simulink model "Pend"  (Simulink 7.4)
settings: Solver=ode45  StartTime=0.0  StopTime=10.0  RelTol=1e-3
libraries: mblibv1 x10
settings Model: Creator=marsryu  LastModifiedBy=marsryu
settings SimMechanicsCC: VisOnUpdateDiagram=on  VisDuringSimulation=on

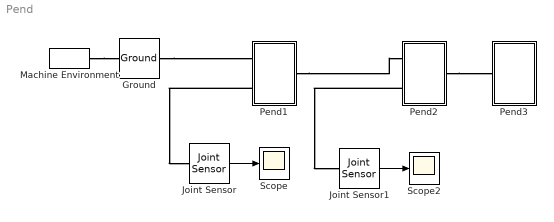
== system Pend ==
  Ground : mblibv1/Bodies/Ground  DialogController=MECH.DynMechDlgSource  SystemSampleTime=-1  UpdateFromCAD=off  LeftPortType=env  RightPortType=workingframe  PhysicalDomain=Mechanical  DialogClass=GroundBlock  CoordPosition=[0 0 0]  CoordPositionUnits=m  StateVectorMgrId=-1  MachineId=[0 0]  ShowEnvPort=on
  Joint Sensor : mblibv1/Sensors &  Actuators/Joint Sensor  DialogController=MECH.DynMechDlgSource  SystemSampleTime=-1  UpdateFromCAD=off  PhysicalDomain=Mechanical  PortType=blob  Muxed=off  Pose=off  Angle=on  AngleUnits=deg  ArcVelocity=off  ArcVelocityUnits=deg/s  ArcAcceleration=off  ArcAccelerationUnits=deg/s^2  CoordPosition=on  CoordPositionUnits=m  Velocity=off  VelocityUnits=m/s  Acceleration=off  AccelerationUnits=m/s^2  Quaternion=on  QuaternionDT=off  QuaternionDDT=off  QuaternionUnits=off  OutputVector=[1]  ActiveIO=on  Width=1  DialogClass=MechanicalSensorBlock  Primitive=R1  Force=off  ForceUnits=N  Torque=off  TorqueUnits=N*m  ReferenceFrame=Absolute (World)  ReactionSensedSide=Base  ReactionReferenceFrame=Absolute (World)  ReactionForce=off  ReactionForceUnits=N  ReactionMoment=off  ReactionMomentUnits=N*m
  Joint Sensor1 : mblibv1/Sensors &  Actuators/Joint Sensor  DialogController=MECH.DynMechDlgSource  SystemSampleTime=-1  UpdateFromCAD=off  PhysicalDomain=Mechanical  PortType=blob  Muxed=on  Pose=off  Angle=on  AngleUnits=deg  ArcVelocity=off  ArcVelocityUnits=deg/s  ArcAcceleration=off  ArcAccelerationUnits=deg/s^2  CoordPosition=on  CoordPositionUnits=m  Velocity=off  VelocityUnits=m/s  Acceleration=off  AccelerationUnits=m/s^2  Quaternion=on  QuaternionDT=off  QuaternionDDT=off  QuaternionUnits=off  OutputVector=[1]  ActiveIO=on  Width=1  DialogClass=MechanicalSensorBlock  Primitive=R1  Force=off  ForceUnits=N  Torque=off  TorqueUnits=N*m  ReferenceFrame=Absolute (World)  ReactionSensedSide=Base  ReactionReferenceFrame=Absolute (World)  ReactionForce=off  ReactionForceUnits=N  ReactionMoment=off  ReactionMomentUnits=N*m
  Machine Environment : mblibv1/Bodies/Machine Environment  DialogController=MECH.DialogSource  SystemSampleTime=-1  PortType=env  PhysicalDomain=Mechanical  DialogTemplateClass=MECH.MachineEnvironment  SyncWhenCopied=off  Gravity=[0 -9.81 0]  GravityUnits=m/s^2  GravityAsSignal=off  Dimensionality=Auto-detect  AnalysisType=Forward dynamics  LinearAssemblyTolerance=1e-3  LinearAssemblyToleranceUnits=m  AngularAssemblyTolerance=1e-3  AngularAssemblyToleranceUnits=rad  ConstraintSolverType=Stabilizing  ConstraintRelTolerance=1e-4  ConstraintAbsTolerance=1e-4  UseRobustSingularityHandling=off  RedundancyAnalysisToleranceType=Automatically select tolerance  RedundancyAnalysisTolerance=1e-14  StatePerturbationType=Fixed  PerturbationSize=1e-5  VisualizeMachine=on  BodyVisualizationType=Use model default body geometries  BodyColorSelMode=Use model default  DefaultBodyColor=[1 0 0]
  Pend1 : Subsystem
  Pend2 : Subsystem
  Pend3 : Subsystem
  Scope : Scope
  Scope2 : Scope
      settings: SaveName=ScopeData2
  wires:
  Joint Sensor/1 -> Scope/1
  Joint Sensor1/1 -> Scope2/1
  connections:
  Ground/RConn1 -- Pend1/LConn1
  Machine Environment/RConn1 -- Ground/LConn1
  Pend1/LConn2 -- Joint Sensor/LConn1
  Pend1/RConn1 -- Pend2/LConn1
  Pend2/RConn1 -- Pend3/LConn1
  Pend2/LConn2 -- Joint Sensor1/LConn1

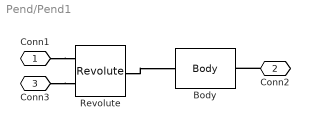
== system Pend/Pend1 ==
  Body : mblibv1/Bodies/Body  DialogController=MECH.DynMechDlgSource  PhysicalDomain=mechanical  SubClassName=Unknown  LeftPortType=workingframe  RightPortType=workingframe  LConnTagsString=CS1  RConnTagsString=CS2  UpdateFromCAD=off  DialogClass=MechanicalBodyBlock  Mass=2472  MassUnits=g  InertiaUnits=g*cm^2  Inertia=diag([206e4,1236,206e4])  Shape=Cylinder  ShapeDims=[1 1]  ShapeUnits=m  ShapeUse=false  Density=1  DensityUnits=kg/m^3  DensityUse=false  GraphicsMode=MACHINE_DEFAULT  GraphicsFileName=C:\Users\marsryu\Desktop\ParallelFrame_Down_Back.stl  BodyColorSelMode=MACHINE_DEFAULT  BodyColor=[1 0 0]  AttachedToCS=CG  CG=Left$CG$[35.36 -35.36 0]$WORLD$WORLD$cm$[0 0 90]$Euler X-Y-Z$deg$WORLD$false$none  WorkingFrames=Left$CS1$[0 0 0]$World$World$cm$[0 0 0]$Euler X-Y-Z$deg$WORLD$true$none#Right$CS2$[70.71 -70.71 0]$World$World$cm$[0 0 0]$Euler X-Y-Z$deg$WORLD$true$none  CGPos=[35.36 -35.36 0]  CGRot=[0 0 90]  CS0Pos=[]  CS0Rot=[]  CS1Pos=[0 0 0]  CS1Rot=[0 0 0]  CS2Pos=[70.71 -70.71 0]  CS2Rot=[0 0 0]  CS3Pos=[]  CS3Rot=[]  CS4Pos=[]  CS4Rot=[]  CS5Pos=[]  CS5Rot=[]  CS6Pos=[]  CS6Rot=[]  CS7Pos=[]  CS7Rot=[]  CS8Pos=[]  CS8Rot=[]  CS9Pos=[]  CS9Rot=[]  CS10Pos=[]  CS10Rot=[]  CS11Pos=[]  CS11Rot=[]  CS12Pos=[]  CS12Rot=[]  CS13Pos=[]  CS13Rot=[]  CS14Pos=[]  CS14Rot=[]  CS15Pos=[]  CS15Rot=[]  CS16Pos=[]  CS16Rot=[]  CS17Pos=[]  CS17Rot=[]  CS18Pos=[]  CS18Rot=[]  CS19Pos=[]  CS19Rot=[]  CS20Pos=[]  CS20Rot=[]
  Revolute : mblibv1/Joints/Revolute  DialogController=MECH.DynMechDlgSource  PhysicalDomain=mechanical  SubClassName=Unknown  LeftPortType=blob  RightPortType=blob  LConnTagsString=__newl0|SA1  RConnTagsString=__newr0  UpdateFromCAD=off  NumSAPorts=1  CutJoint=off  MarkAsCut=off  Primitives=prismatic  PrimitiveProps=R1$World$[0 0 1]$revolute  DialogClass=JointBlock  R1Axis=[0 0 1]
  Conn1 : PMIOPort  Port=1  Side=Left
  Conn2 : PMIOPort  Port=2  Side=Right
  Conn3 : PMIOPort  Port=3  Side=Left
  connections:
  Revolute/RConn1 -- Body/LConn1
  Conn1/RConn1 -- Revolute/LConn1
  Conn2/RConn1 -- Body/RConn1
  Conn3/RConn1 -- Revolute/LConn2

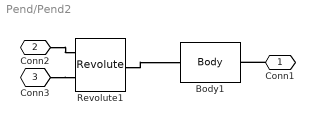
== system Pend/Pend2 ==
  Body1 : mblibv1/Bodies/Body  DialogController=MECH.DynMechDlgSource  PhysicalDomain=mechanical  SubClassName=Unknown  LeftPortType=workingframe  RightPortType=workingframe  LConnTagsString=CS1  RConnTagsString=CS2  UpdateFromCAD=off  DialogClass=MechanicalBodyBlock  Mass=2472  MassUnits=g  InertiaUnits=g*cm^2  Inertia=diag([206e4,1236,206e4])  Shape=Cylinder  ShapeDims=[1 1]  ShapeUnits=m  ShapeUse=false  Density=1  DensityUnits=kg/m^3  DensityUse=false  GraphicsMode=MACHINE_DEFAULT  BodyColorSelMode=MACHINE_DEFAULT  BodyColor=[1 0 0]  AttachedToCS=CG  CG=Left$CG$[0 -50 0]$CS1$CS1$cm$[0 0 0]$Euler X-Y-Z$deg$CS1$false$none  WorkingFrames=Left$CS1$[0 0 0]$Adjoining$Adjoining$cm$[0 0 45]$Euler X-Y-Z$deg$WORLD$true$none#Right$CS2$[0 -100 0]$CS1$CS1$cm$[0 0 0]$Euler X-Y-Z$deg$WORLD$true$none  CGPos=[0 -50 0]  CGRot=[0 0 0]  CS0Pos=[]  CS0Rot=[]  CS1Pos=[0 0 0]  CS1Rot=[0 0 45]  CS2Pos=[0 -100 0]  CS2Rot=[0 0 0]  CS3Pos=[]  CS3Rot=[]  CS4Pos=[]  CS4Rot=[]  CS5Pos=[]  CS5Rot=[]  CS6Pos=[]  CS6Rot=[]  CS7Pos=[]  CS7Rot=[]  CS8Pos=[]  CS8Rot=[]  CS9Pos=[]  CS9Rot=[]  CS10Pos=[]  CS10Rot=[]  CS11Pos=[]  CS11Rot=[]  CS12Pos=[]  CS12Rot=[]  CS13Pos=[]  CS13Rot=[]  CS14Pos=[]  CS14Rot=[]  CS15Pos=[]  CS15Rot=[]  CS16Pos=[]  CS16Rot=[]  CS17Pos=[]  CS17Rot=[]  CS18Pos=[]  CS18Rot=[]  CS19Pos=[]  CS19Rot=[]  CS20Pos=[]  CS20Rot=[]
  Revolute1 : mblibv1/Joints/Revolute  DialogController=MECH.DynMechDlgSource  PhysicalDomain=mechanical  SubClassName=Unknown  LeftPortType=blob  RightPortType=blob  LConnTagsString=__newl0|SA1  RConnTagsString=__newr0  UpdateFromCAD=off  NumSAPorts=1  CutJoint=off  MarkAsCut=off  Primitives=prismatic  PrimitiveProps=R1$World$[0 0 1]$revolute  DialogClass=JointBlock  R1Axis=[0 0 1]
  Conn1 : PMIOPort  Port=1  Side=Right
  Conn2 : PMIOPort  Port=2  Side=Left
  Conn3 : PMIOPort  Port=3  Side=Left
  connections:
  Revolute1/RConn1 -- Body1/LConn1
  Conn1/RConn1 -- Body1/RConn1
  Conn2/RConn1 -- Revolute1/LConn1
  Conn3/RConn1 -- Revolute1/LConn2

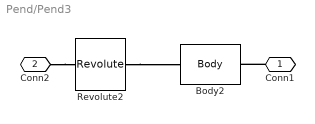
== system Pend/Pend3 ==
  Body2 : mblibv1/Bodies/Body  DialogController=MECH.DynMechDlgSource  PhysicalDomain=mechanical  SubClassName=Unknown  LeftPortType=workingframe  RightPortType=workingframe  LConnTagsString=CS1  RConnTagsString=CS2  UpdateFromCAD=off  DialogClass=MechanicalBodyBlock  Mass=2472  MassUnits=g  InertiaUnits=g*cm^2  Inertia=diag([206e4,1236,206e4])  Shape=Cylinder  ShapeDims=[1 1]  ShapeUnits=m  ShapeUse=false  Density=1  DensityUnits=kg/m^3  DensityUse=false  GraphicsMode=MACHINE_DEFAULT  BodyColorSelMode=MACHINE_DEFAULT  BodyColor=[1 0 0]  AttachedToCS=CG  CG=Left$CG$[0 -50 0]$CS1$CS1$cm$[0 0 0]$Euler X-Y-Z$deg$CS1$false$none  WorkingFrames=Left$CS1$[0 0 0]$Adjoining$Adjoining$cm$[0 0 45]$Euler X-Y-Z$deg$WORLD$true$none#Right$CS2$[0 -100 0]$CS1$CS1$cm$[0 0 0]$Euler X-Y-Z$deg$WORLD$true$none  CGPos=[0 -50 0]  CGRot=[0 0 0]  CS0Pos=[]  CS0Rot=[]  CS1Pos=[0 0 0]  CS1Rot=[0 0 45]  CS2Pos=[0 -100 0]  CS2Rot=[0 0 0]  CS3Pos=[]  CS3Rot=[]  CS4Pos=[]  CS4Rot=[]  CS5Pos=[]  CS5Rot=[]  CS6Pos=[]  CS6Rot=[]  CS7Pos=[]  CS7Rot=[]  CS8Pos=[]  CS8Rot=[]  CS9Pos=[]  CS9Rot=[]  CS10Pos=[]  CS10Rot=[]  CS11Pos=[]  CS11Rot=[]  CS12Pos=[]  CS12Rot=[]  CS13Pos=[]  CS13Rot=[]  CS14Pos=[]  CS14Rot=[]  CS15Pos=[]  CS15Rot=[]  CS16Pos=[]  CS16Rot=[]  CS17Pos=[]  CS17Rot=[]  CS18Pos=[]  CS18Rot=[]  CS19Pos=[]  CS19Rot=[]  CS20Pos=[]  CS20Rot=[]
  Revolute2 : mblibv1/Joints/Revolute  DialogController=MECH.DynMechDlgSource  PhysicalDomain=mechanical  SubClassName=Unknown  LeftPortType=blob  RightPortType=blob  LConnTagsString=__newl0  RConnTagsString=__newr0  UpdateFromCAD=off  NumSAPorts=0  CutJoint=off  MarkAsCut=off  Primitives=prismatic  PrimitiveProps=R1$World$[0 0 1]$revolute  DialogClass=JointBlock  R1Axis=[0 0 1]
  Conn1 : PMIOPort  Port=1  Side=Right
  Conn2 : PMIOPort  Port=2  Side=Left
  connections:
  Revolute2/RConn1 -- Body2/LConn1
  Conn1/RConn1 -- Body2/RConn1
  Conn2/RConn1 -- Revolute2/LConn1
